simulink model "Sim_Demo"  (R2022a)
settings: Solver=VariableStepAuto  StartTime=0.0  StopTime=15  RelTol=1e-3
libraries: autolibshared x1
settings Model: Creator=YZD  LastModifiedBy=YZD

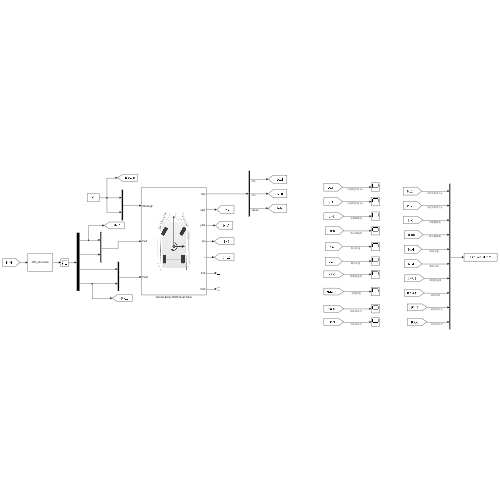
[thumbnail: Simulink's stored preview of the top-level diagram]
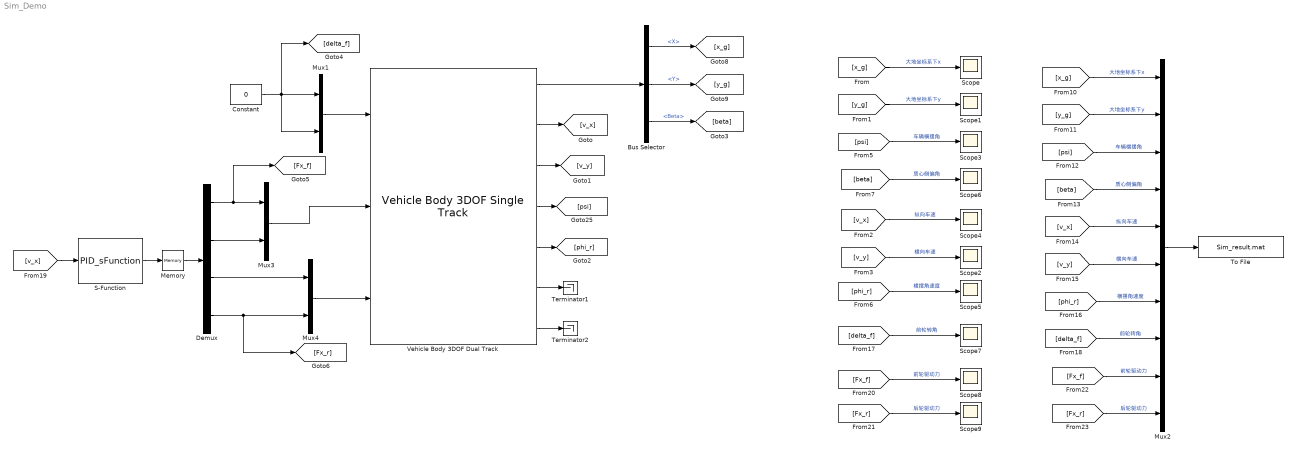
== system Sim_Demo ==
  Bus Selector : BusSelector  OutputSignals=InertFrm.Cg.Disp.X,InertFrm.Cg.Disp.Y,BdyFrm.Cg.Ang.Beta
  Constant : Constant  Value=0
  Demux : Demux
  Memory : Memory
  Mux1 : Mux  Inputs=2
  Mux2 : Mux  Inputs=10
  Mux3 : Mux  Inputs=2
  Mux4 : Mux  Inputs=2
  S-Function : S-Function  FunctionName=PID_sFunction  SFunctionDeploymentMode=off  EnableBusSupport=off
  Scope{,1..9} (10 alike) : Scope
  Terminator1 : Terminator
  Terminator2 : Terminator
  To File : ToFile  Filename=Sim_result.mat  MatrixName=out  SaveFormat=Timeseries  SampleTime=0.01
  Vehicle Body 3DOF Dual Track : autolibshared/Vehicle Body 3DOF Single Track  trackMode=Dual  inputMode=External longitudinal forces  frontSteerMode=on  rearSteerMode=off  windMode=off  muMode=off  extFMode=off  extMMode=off  htchFMode=off  htchMMode=off  extXo=off  extpsio=off  extxdoto=off  extro=off  extYo=off  extTamb=off  extydoto=off  aMode=2  NF=2  NR=2  m=2000  a=1.4  b=1.6  h=0.35  dh=1  hh=0.2  X_o=0  xdot_o=5  CalphaMode=off  sigmaMode=on  d=0  hl=0  w=[1.4,1.4]  Cy_f=12e3  Cy_r=11e3  sigma_f=.1  sigma_r=.1  alpha_f_brk=[-.1 .1]  Cy_f_data=[-9e3 9e3]  alpha_r_brk=[-.1 .1]  Cy_r_data=[-9e3 9e3]  Y_o=0  ydot_o=0  Izz=4000  psi_o=0  r_o=0  Af=2  Cd=.3  Cl=.1  Cpm=.1  beta_w=[0 0.01:0.01:0.3]  Cs=[0:0.03:0.9]  Cym=[0 1e-6:0.01:0.3]  Pabs=101325  Tair=273  g=9.81  mu=1  xdot_tol=.01  Fznom=5000  Fxtire_sat=7e4  Fytire_sat=7e4  longOff=0  latOff=0  vertOff=0  wrapAng=off
      settings: SourceProductBaseCode=PW,DR,MT,VE
  wires:
  Vehicle Body 3DOF Dual Track/4 -> [psi]
  Vehicle Body 3DOF Dual Track/2 -> [v_x]
  Vehicle Body 3DOF Dual Track/3 -> [v_y]
  Vehicle Body 3DOF Dual Track/5 -> [phi_r]
  S-Function/1 -> Memory/1
  Memory/1 -> Demux/1
  Vehicle Body 3DOF Dual Track/1 -> Bus Selector/1
  Bus Selector/3 -> [beta]  "<Beta>"
  Bus Selector/1 -> [x_g]  "<X>"
  Bus Selector/2 -> [y_g]  "<Y>"
  Vehicle Body 3DOF Dual Track/6 -> Terminator1/1
  Vehicle Body 3DOF Dual Track/7 -> Terminator2/1
  [x_g] -> Scope/1  "大地坐标系下x"
  [y_g] -> Scope1/1  "大地坐标系下y"
  [psi] -> Scope3/1  "车辆横摆角"
  [v_y] -> Scope2/1  "横向车速"
  [v_x] -> Scope4/1  "纵向车速"
  [phi_r] -> Scope5/1  "横摆角速度"
  [beta] -> Scope6/1  "质心侧偏角"
  [beta] -> Mux2/4  "质心侧偏角"
  [psi] -> Mux2/3  "车辆横摆角"
  [y_g] -> Mux2/2  "大地坐标系下y"
  [x_g] -> Mux2/1  "大地坐标系下x"
  [phi_r] -> Mux2/7  "横摆角速度"
  [v_x] -> Mux2/5  "纵向车速"
  [v_y] -> Mux2/6  "横向车速"
  Mux2/1 -> To File/1
  [delta_f] -> Scope7/1  "前轮转角"
  [delta_f] -> Mux2/8  "前轮转角"
  Mux1/1 -> Vehicle Body 3DOF Dual Track/1
  Mux3/1 -> Vehicle Body 3DOF Dual Track/2
  Mux4/1 -> Vehicle Body 3DOF Dual Track/3
  Demux/2 -> Mux3/2
  Demux/1 -> Mux3/1, [Fx_f]
  Demux/3 -> Mux4/1
  Demux/4 -> [Fx_r], Mux4/2
  [Fx_f] -> Scope8/1  "前轮驱动力"
  [Fx_r] -> Scope9/1  "后轮驱动力"
  [Fx_r] -> Mux2/10  "后轮驱动力"
  [Fx_f] -> Mux2/9  "前轮驱动力"
  [v_x] -> S-Function/1
  Constant/1 -> Mux1/2, [delta_f], Mux1/1
